simulink model "P1_Part2_Option2 (2)"  (R2023b)
settings: Solver=VariableStepAuto  StartTime=0.0  StopTime=25  RelTol=1e-3
values from neighbouring files (symbols this model uses):
  b1 = 1    [Project1_Part2.m]
  b2 = 1    [Project1_Part2.m]
  J1 = 100    [Project1_Part2.m]
  J2 = 1    [Project1_Part2.m]
  T_app = index1    [Project1_Part2.m]
settings Model: Creator=luker  LastModifiedBy=luker

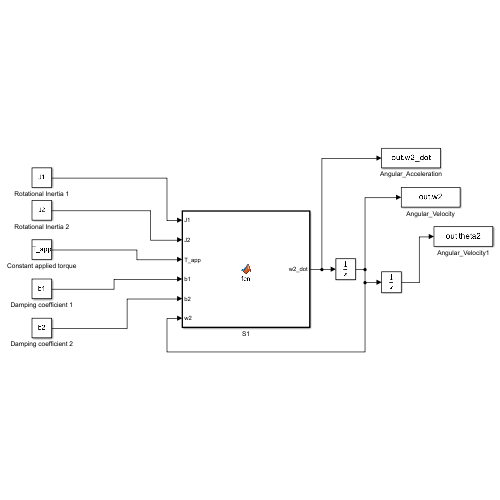
[thumbnail: Simulink's stored preview of the top-level diagram]
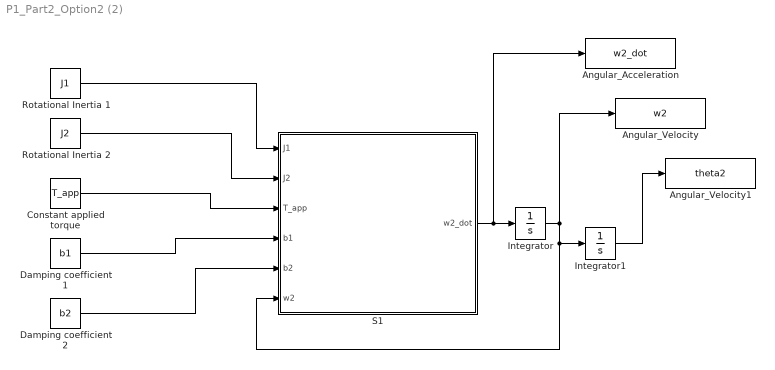
== system P1_Part2_Option2 (2) ==
  Angular_Acceleration : ToWorkspace  VariableName=w2_dot  SaveFormat=Timeseries  SampleTime=-1
  Angular_Velocity : ToWorkspace  VariableName=w2  SaveFormat=Timeseries  SampleTime=-1
  Angular_Velocity1 : ToWorkspace  VariableName=theta2  SaveFormat=Timeseries  SampleTime=-1
  Constant applied torque : Constant  Value=T_app
  Damping coefficient 1 : Constant  Value=b1
  Damping coefficient 2 : Constant  Value=b2
  Integrator : Integrator  UpperSaturationLimit=<binary blob, 304 chars, not shown>  LowerSaturationLimit=<binary blob, 305 chars, not shown>
  Integrator1 : Integrator  UpperSaturationLimit=<binary blob, 304 chars, not shown>  LowerSaturationLimit=<binary blob, 305 chars, not shown>
  Rotational Inertia 1 : Constant  Value=J1
  Rotational Inertia 2 : Constant  Value=J2
  S1 : MATLAB Function  TreatAsAtomicUnit=on
  wires:
  Rotational Inertia 1/1 -> S1/1(J1)
  Rotational Inertia 2/1 -> S1/2(J2)
  Damping coefficient 1/1 -> S1/4(b1)
  Damping coefficient 2/1 -> S1/5(b2)
  Constant applied torque/1 -> S1/3(T_app)
  S1/1(w2_dot) -> Angular_Acceleration/1, Integrator/1
  Integrator/1 -> S1/6(w2), Integrator1/1, Angular_Velocity/1
  Integrator1/1 -> Angular_Velocity1/1

== matlab function P1_Part2_Option2 (2)/S1 ==
  data: J1 input; J2 input; w2_dot output; T_app input; b1 input; b2 input; w2 input
function w2_dot = fcn(J1, J2, T_app, b1, b2, w2)
% GIVENS:
% J1
% B1
% J2
% B2
% T_app - Constant Applied Torque
% FOR OPTION 1:
% k

w2_dot = (1/(J1+J2))*(T_app-(b1+b2)*w2);
end
